simulink model "TestCase_Arch_Car_mapping"  (R2016b)
settings: Solver=FixedStepAuto  StartTime=0.0  StopTime=10.0  RelTol=1e-3
model workspace: external: MAT-File TestCase_Arch_Car_mapping.mat (data not in the file)
libraries: libTLAsserts x4
settings Model: Creator=NEATdemo  LastModifiedBy=NEATdemo

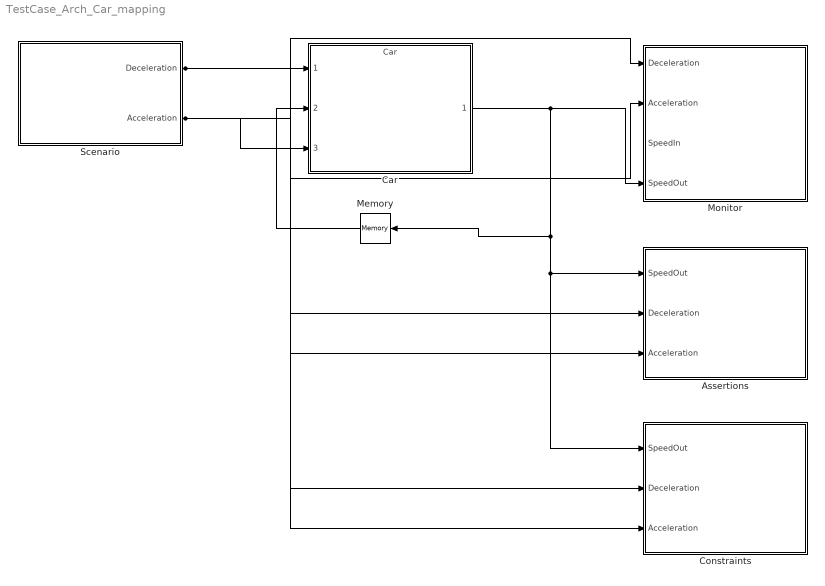
== system TestCase_Arch_Car_mapping ==
  Assertions : Subsystem
  Car : ModelReference  ModelNameDialog=Car  SimulationMode=Normal  ModelReferenceVersion=1.9
  Constraints : Subsystem
  Memory : Memory
  Monitor : Subsystem
  Scenario : Subsystem
  wires:
  Scenario/1(Deceleration) -> Car/1, Monitor/1(Deceleration), Assertions/2(Deceleration), Constraints/2(Deceleration)
  Scenario/2(Acceleration) -> Car/3, Monitor/2(Acceleration), Assertions/3(Acceleration), Constraints/3(Acceleration)
  Car/1 -> Memory/1, Assertions/1(SpeedOut), Constraints/1(SpeedOut), Monitor/4(SpeedOut)
  Memory/1 -> Car/2

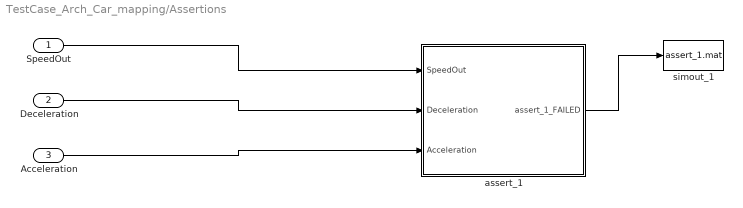
== system TestCase_Arch_Car_mapping/Assertions ==
  SpeedOut : Inport
  Deceleration : Inport  Port=2
  Acceleration : Inport  Port=3
  assert_1 : Subsystem
  simout_1 : ToFile  Filename=assert_1.mat  MatrixName=assert_1  SaveFormat=Timeseries
  wires:
  SpeedOut/1 -> assert_1/1(SpeedOut)
  Deceleration/1 -> assert_1/2(Deceleration)
  Acceleration/1 -> assert_1/3(Acceleration)
  assert_1/1(assert_1_FAILED) -> simout_1/1

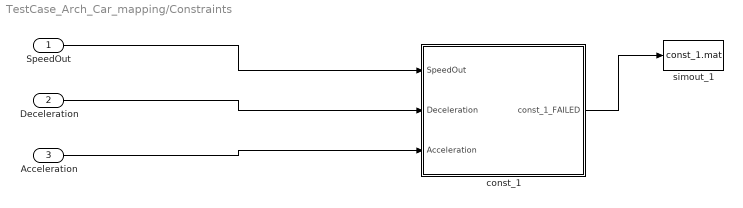
== system TestCase_Arch_Car_mapping/Constraints ==
  SpeedOut : Inport
  Deceleration : Inport  Port=2
  Acceleration : Inport  Port=3
  const_1 : Subsystem
  simout_1 : ToFile  Filename=const_1.mat  MatrixName=const_1  SaveFormat=Timeseries
  wires:
  SpeedOut/1 -> const_1/1(SpeedOut)
  Deceleration/1 -> const_1/2(Deceleration)
  Acceleration/1 -> const_1/3(Acceleration)
  const_1/1(const_1_FAILED) -> simout_1/1

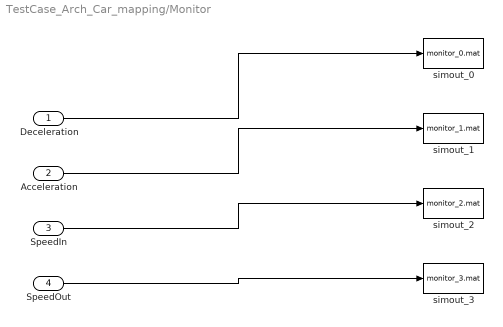
== system TestCase_Arch_Car_mapping/Monitor ==
  Deceleration : Inport
  Acceleration : Inport  Port=2
  SpeedIn : Inport  Port=3
  SpeedOut : Inport  Port=4
  simout_0 : ToFile  Filename=monitor_0.mat  MatrixName=Deceleration  SaveFormat=Timeseries
  simout_1 : ToFile  Filename=monitor_1.mat  MatrixName=Acceleration  SaveFormat=Timeseries
  simout_2 : ToFile  Filename=monitor_2.mat  MatrixName=SpeedIn  SaveFormat=Timeseries
  simout_3 : ToFile  Filename=monitor_3.mat  MatrixName=SpeedOut  SaveFormat=Timeseries
  wires:
  Deceleration/1 -> simout_0/1
  Acceleration/1 -> simout_1/1
  SpeedIn/1 -> simout_2/1
  SpeedOut/1 -> simout_3/1

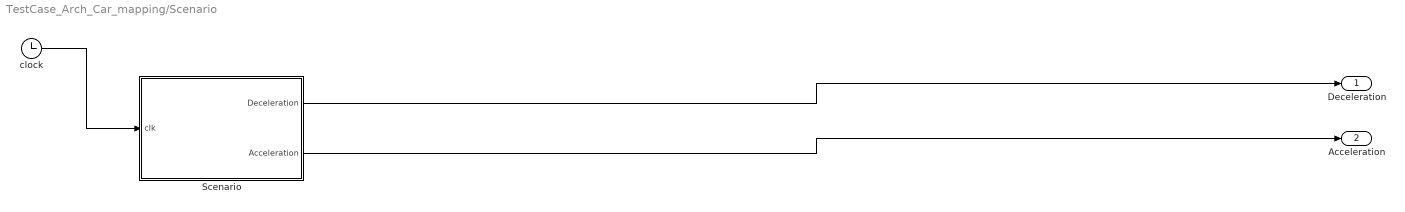
== system TestCase_Arch_Car_mapping/Scenario ==
  Scenario : Stateflow chart  TreatAsAtomicUnit=on
  clock : Clock
  Deceleration : Outport
  Acceleration : Outport  Port=2
  wires:
  Scenario/1(Deceleration) -> Deceleration/1
  Scenario/2(Acceleration) -> Acceleration/1
  clock/1 -> Scenario/1(clk)

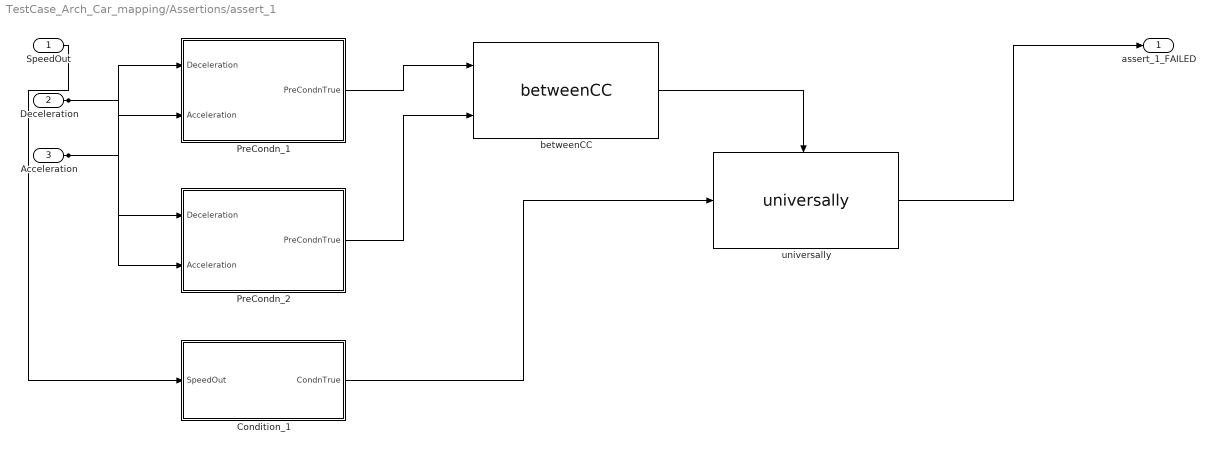
== system TestCase_Arch_Car_mapping/Assertions/assert_1 ==
  SpeedOut : Inport
  Deceleration : Inport  Port=2
  Acceleration : Inport  Port=3
  Condition_1 : Subsystem
  PreCondn_1 : Subsystem
  PreCondn_2 : Subsystem
  betweenCC : libTLAsserts/betweenCC
  universally : libTLAsserts/universally
  assert_1_FAILED : Outport
  wires:
  Deceleration/1 -> PreCondn_1/1(Deceleration), PreCondn_2/1(Deceleration)
  Acceleration/1 -> PreCondn_1/2(Acceleration), PreCondn_2/2(Acceleration)
  SpeedOut/1 -> Condition_1/1(SpeedOut)
  PreCondn_1/1(PreCondnTrue) -> betweenCC/1
  PreCondn_2/1(PreCondnTrue) -> betweenCC/2
  Condition_1/1(CondnTrue) -> universally/1
  betweenCC/1 -> universally/Enable
  universally/1 -> assert_1_FAILED/1

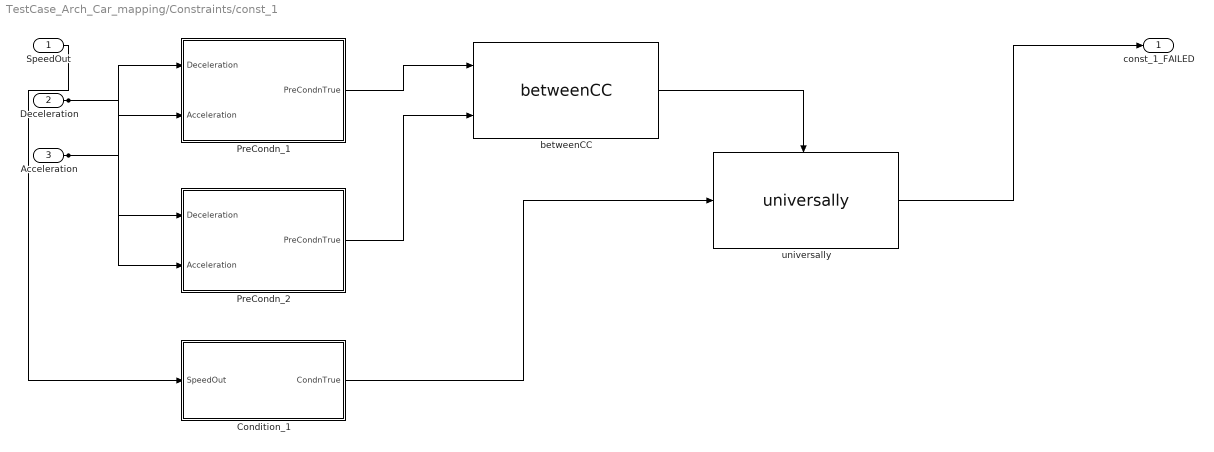
== system TestCase_Arch_Car_mapping/Constraints/const_1 ==
  SpeedOut : Inport
  Deceleration : Inport  Port=2
  Acceleration : Inport  Port=3
  Condition_1 : Subsystem
  PreCondn_1 : Subsystem
  PreCondn_2 : Subsystem
  betweenCC : libTLAsserts/betweenCC
  universally : libTLAsserts/universally
  const_1_FAILED : Outport
  wires:
  Deceleration/1 -> PreCondn_1/1(Deceleration), PreCondn_2/1(Deceleration)
  Acceleration/1 -> PreCondn_1/2(Acceleration), PreCondn_2/2(Acceleration)
  SpeedOut/1 -> Condition_1/1(SpeedOut)
  PreCondn_1/1(PreCondnTrue) -> betweenCC/1
  PreCondn_2/1(PreCondnTrue) -> betweenCC/2
  Condition_1/1(CondnTrue) -> universally/1
  betweenCC/1 -> universally/Enable
  universally/1 -> const_1_FAILED/1

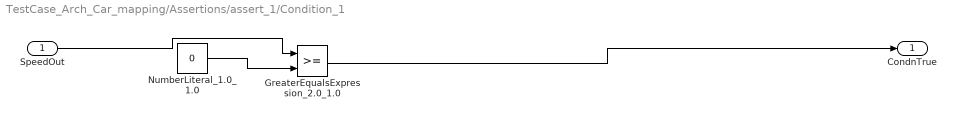
== system TestCase_Arch_Car_mapping/Assertions/assert_1/Condition_1 ==
  SpeedOut : Inport
  GreaterEqualsExpression_2.0_1.0 : RelationalOperator  OutDataTypeStr=boolean  RndMeth=Simplest
  NumberLiteral_1.0_1.0 : Constant  Value=0
  CondnTrue : Outport
  wires:
  SpeedOut/1 -> GreaterEqualsExpression_2.0_1.0/1
  NumberLiteral_1.0_1.0/1 -> GreaterEqualsExpression_2.0_1.0/2
  GreaterEqualsExpression_2.0_1.0/1 -> CondnTrue/1

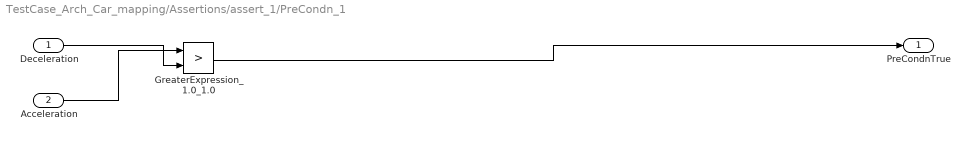
== system TestCase_Arch_Car_mapping/Assertions/assert_1/PreCondn_1 ==
  Deceleration : Inport
  Acceleration : Inport  Port=2
  GreaterExpression_1.0_1.0 : RelationalOperator  Operator=>  OutDataTypeStr=boolean  RndMeth=Simplest
  PreCondnTrue : Outport
  wires:
  Acceleration/1 -> GreaterExpression_1.0_1.0/1
  Deceleration/1 -> GreaterExpression_1.0_1.0/2
  GreaterExpression_1.0_1.0/1 -> PreCondnTrue/1

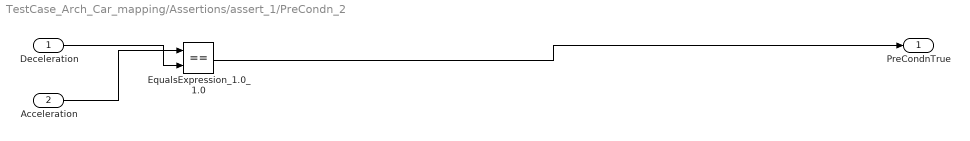
== system TestCase_Arch_Car_mapping/Assertions/assert_1/PreCondn_2 ==
  Deceleration : Inport
  Acceleration : Inport  Port=2
  EqualsExpression_1.0_1.0 : RelationalOperator  Operator===  OutDataTypeStr=boolean  RndMeth=Simplest
  PreCondnTrue : Outport
  wires:
  Acceleration/1 -> EqualsExpression_1.0_1.0/1
  Deceleration/1 -> EqualsExpression_1.0_1.0/2
  EqualsExpression_1.0_1.0/1 -> PreCondnTrue/1

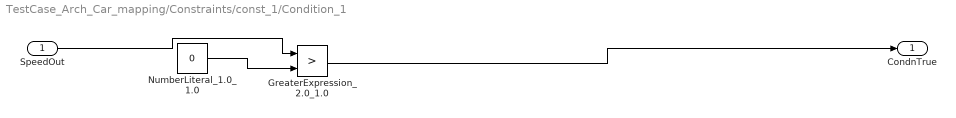
== system TestCase_Arch_Car_mapping/Constraints/const_1/Condition_1 ==
  SpeedOut : Inport
  GreaterExpression_2.0_1.0 : RelationalOperator  Operator=>  OutDataTypeStr=boolean  RndMeth=Simplest
  NumberLiteral_1.0_1.0 : Constant  Value=0
  CondnTrue : Outport
  wires:
  SpeedOut/1 -> GreaterExpression_2.0_1.0/1
  NumberLiteral_1.0_1.0/1 -> GreaterExpression_2.0_1.0/2
  GreaterExpression_2.0_1.0/1 -> CondnTrue/1

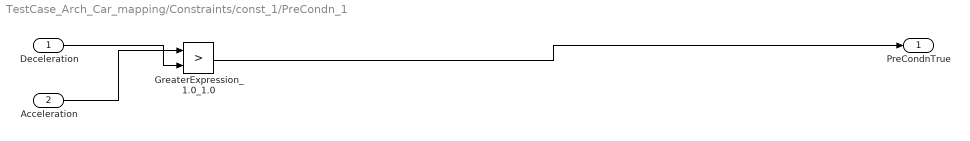
== system TestCase_Arch_Car_mapping/Constraints/const_1/PreCondn_1 ==
  Deceleration : Inport
  Acceleration : Inport  Port=2
  GreaterExpression_1.0_1.0 : RelationalOperator  Operator=>  OutDataTypeStr=boolean  RndMeth=Simplest
  PreCondnTrue : Outport
  wires:
  Acceleration/1 -> GreaterExpression_1.0_1.0/1
  Deceleration/1 -> GreaterExpression_1.0_1.0/2
  GreaterExpression_1.0_1.0/1 -> PreCondnTrue/1

== system TestCase_Arch_Car_mapping/Constraints/const_1/PreCondn_2 ==
  Deceleration : Inport
  Acceleration : Inport  Port=2
  EqualsExpression_1.0_1.0 : RelationalOperator  Operator===  OutDataTypeStr=boolean  RndMeth=Simplest
  PreCondnTrue : Outport
  wires:
  Acceleration/1 -> EqualsExpression_1.0_1.0/1
  Deceleration/1 -> EqualsExpression_1.0_1.0/2
  EqualsExpression_1.0_1.0/1 -> PreCondnTrue/1

== stateflow chart TestCase_Arch_Car_mapping/Scenario/Scenario ==
  state Act_Car_Step1
    entry: Deceleration = 10;
    entry: Acceleration = Deceleration;
  state Act_Car_Step2
    entry: Acceleration = 110;
    entry: Act_Car_Step2_stpClk = clk;
  state Act_Car_Step3
    entry: Acceleration = Deceleration;
  state Act_Car_Step4
    entry: Act_Car_Step4_stpClk = clk;
  (default) -> Act_Car_Step1
  Act_Car_Step1 -> Act_Car_Step2
  Act_Car_Step2 -> Act_Car_Step3 : [clk - Act_Car_Step2_stpClk >= 5]
  Act_Car_Step3 -> Act_Car_Step4
  data: clk input; Deceleration output; Acceleration output; Act_Car_Step2_stpClk local; Act_Car_Step4_stpClk local
